simulink model "simulator_real"  (R2025b)
settings: Solver=ode15s  StartTime=0.0  StopTime=50  FixedStep=0.001  RelTol=1e-3
InitFcn:
  | run('rocket3d_params.m')
values from neighbouring files (symbols this model uses):
  A_e = pi*(d_e/2)^2    (= 0.000346360590058)    [rocket3d_params.m]
  A_rocket = pi*(d_rocket/2)^2    (= 0.006647610055)    [rocket3d_params.m]
  beta_poly = 1.31    [rocket3d_params.m]
  C_d_air = 0.90    (= 0.9)    [rocket3d_params.m]
  C_D_drag = 0.25    [rocket3d_params.m]
  C_d_water = 0.85    [rocket3d_params.m]
  CG_dry_body = [0.01289;  0.01855; -0.00576]    [rocket3d_params.m]
  CG_dry_Y = 0.01855    [rocket3d_params.m]
  CG_full_body = [0.01345; -0.10517; -0.00608]    [rocket3d_params.m]
  CG_full_Y = -0.10517    [rocket3d_params.m]
  D = q * A_rocket * Cd0    [aero_func.m]
  gamma_gas = 1.4    [rocket3d_params.m]
  I_dry_vec = [3.0e-3;  5.071e-4; 3.0e-3;  6.928e-7;  2.156e-6; -2.712e-6]    [rocket3d_params.m]
  I_full_vec = [1.1e-2;  1.0e-3;   1.1e-2;  3.14e-5;   2.234e-6; -1.994e-5]    [rocket3d_params.m]
  m_dry_i = 0.269    [rocket3d_params.m]
  m_empty = m_dry_i    (= 0.269)    [rocket3d_params.m]
  m_full = m_dry_i + m_water_0    (= 0.849)    [rocket3d_params.m]
  m_water_0 = 0.580    (= 0.58)    [rocket3d_params.m]
  N = round(t_sim/Ts)    [stability_margin_timehistory.m]
  P_atm = 101325    [rocket3d_params.m]
  P_i = 50*6894.75 + P_atm    (= 446062.5)    [rocket3d_params.m]
  R_gas = 287.05    [rocket3d_params.m]
  rho_air_ext = 1.225    [rocket3d_params.m]
  rho_water = 1000    [rocket3d_params.m]
  T_i = T_celsius + 273.15    (= 298.15)    [rocket3d_params.m]
  Ts = 0.001    [rocket3d_params.m]    (also in stability_margin_timehistory.m)
  V_bottle = 1.5e-3    (= 0.0015)    [rocket3d_params.m]
  V_gas_i = V_bottle - V_water_i    (= 0.00092)    [rocket3d_params.m]
  Y_CP_body = 0.160119 - 0.255    (= -0.094881)    [rocket3d_params.m]
undefined symbols (not defined in the file or in its folder): X, Y, Z
libraries: nesl_utility x14, sm_lib x10
settings Model: Creator=user  LastModifiedBy=user

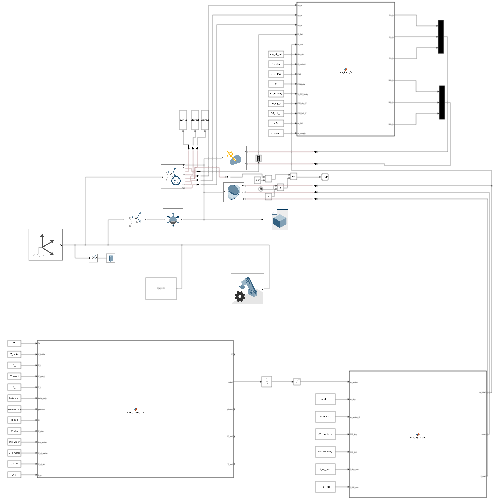
[thumbnail: Simulink's stored preview of the top-level diagram]
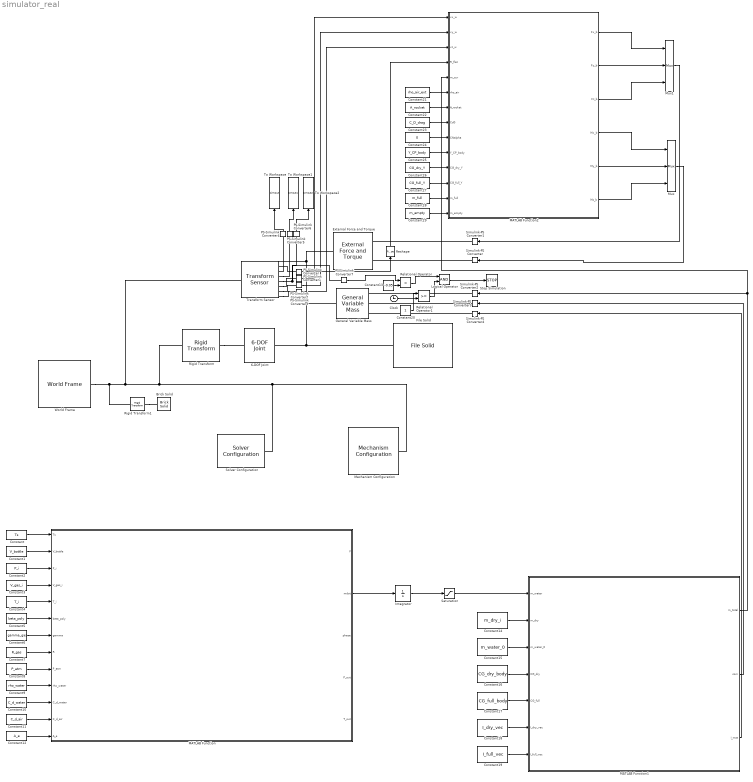
== system simulator_real ==
  6-DOF Joint : sm_lib/Joints/6-DOF Joint  JointMode=Normal  CompositeWrenchDir=FollowerOnBase  CompositeWrenchFrame=BaseFrame  SenseConstraintForce=off  SenseConstraintTorque=off  SenseTotalForce=off  SenseTotalTorque=off  PxPositionTargetSpecify=off  PxPositionTargetPriority=High  PxPositionTargetValue=0  PxPositionTargetValueUnits=m  PxVelocityTargetSpecify=off  PxVelocityTargetPriority=High  PxVelocityTargetValue=0  PxVelocityTargetValueUnits=m/s  PxEquilibriumPosition=0  PxEquilibriumPositionUnits=m  PxSpringStiffness=0  PxSpringStiffnessUnits=N/m  PxDampingCoefficient=0  PxDampingCoefficientUnits=N/(m/s)  PxLowerLimitSpecify=off  PxLowerLimitBound=-1  PxLowerLimitBoundUnits=m  PxLowerLimitStiffness=1e6  PxLowerLimitStiffnessUnits=N/m  PxLowerLimitDamping=1e3  PxLowerLimitDampingUnits=N/(m/s)  PxLowerLimitTransitionRegionWidth=1e-4  PxLowerLimitTransitionRegionWidthUnits=m  PxUpperLimitSpecify=off  PxUpperLimitBound=1  PxUpperLimitBoundUnits=m  PxUpperLimitStiffness=1e6  PxUpperLimitStiffnessUnits=N/m  PxUpperLimitDamping=1e3  PxUpperLimitDampingUnits=N/(m/s)  PxUpperLimitTransitionRegionWidth=1e-4  PxUpperLimitTransitionRegionWidthUnits=m  PxTorqueActuationMode=NoTorque  PxMotionActuationMode=ComputedMotion  PxSensePosition=off  PxSenseVelocity=off  PxSenseAcceleration=off  PxSenseTorqueForce=off  PxSenseLowerLimitTorqueForce=off  PxSenseUpperLimitTorqueForce=off  PyPositionTargetSpecify=off  PyPositionTargetPriority=High  PyPositionTargetValue=0  PyPositionTargetValueUnits=m  PyVelocityTargetSpecify=off  PyVelocityTargetPriority=High  PyVelocityTargetValue=0  PyVelocityTargetValueUnits=m/s  PyEquilibriumPosition=0  PyEquilibriumPositionUnits=m  PySpringStiffness=0  PySpringStiffnessUnits=N/m  PyDampingCoefficient=0  PyDampingCoefficientUnits=N/(m/s)  PyLowerLimitSpecify=off  PyLowerLimitBound=-1  PyLowerLimitBoundUnits=m  PyLowerLimitStiffness=1e6  PyLowerLimitStiffnessUnits=N/m  PyLowerLimitDamping=1e3  PyLowerLimitDampingUnits=N/(m/s)  PyLowerLimitTransitionRegionWidth=1e-4  PyLowerLimitTransitionRegionWidthUnits=m  PyUpperLimitSpecify=off  PyUpperLimitBound=1  PyUpperLimitBoundUnits=m  PyUpperLimitStiffness=1e6  PyUpperLimitStiffnessUnits=N/m  PyUpperLimitDamping=1e3  PyUpperLimitDampingUnits=N/(m/s)  PyUpperLimitTransitionRegionWidth=1e-4  PyUpperLimitTransitionRegionWidthUnits=m  PyTorqueActuationMode=NoTorque  PyMotionActuationMode=ComputedMotion  PySensePosition=off  PySenseVelocity=off  PySenseAcceleration=off  PySenseTorqueForce=off  PySenseLowerLimitTorqueForce=off  PySenseUpperLimitTorqueForce=off  PzPositionTargetSpecify=on  PzPositionTargetPriority=High  PzPositionTargetValue=0.3  PzPositionTargetValueUnits=m  PzVelocityTargetSpecify=off  PzVelocityTargetPriority=High  PzVelocityTargetValue=0  PzVelocityTargetValueUnits=m/s  PzEquilibriumPosition=0  PzEquilibriumPositionUnits=m  PzSpringStiffness=0  PzSpringStiffnessUnits=N/m  PzDampingCoefficient=0  PzDampingCoefficientUnits=N/(m/s)  PzLowerLimitSpecify=off  PzLowerLimitBound=-1  PzLowerLimitBoundUnits=m  PzLowerLimitStiffness=1e6  PzLowerLimitStiffnessUnits=N/m  PzLowerLimitDamping=1e3  PzLowerLimitDampingUnits=N/(m/s)  PzLowerLimitTransitionRegionWidth=1e-4  PzLowerLimitTransitionRegionWidthUnits=m  PzUpperLimitSpecify=off  PzUpperLimitBound=1  PzUpperLimitBoundUnits=m  PzUpperLimitStiffness=1e6  PzUpperLimitStiffnessUnits=N/m  PzUpperLimitDamping=1e3  PzUpperLimitDampingUnits=N/(m/s)  PzUpperLimitTransitionRegionWidth=1e-4  PzUpperLimitTransitionRegionWidthUnits=m  PzTorqueActuationMode=NoTorque  PzMotionActuationMode=ComputedMotion  PzSensePosition=off  PzSenseVelocity=off  PzSenseAcceleration=off  PzSenseTorqueForce=off  PzSenseLowerLimitTorqueForce=off  PzSenseUpperLimitTorqueForce=off  SphPositionTargetSpecify=off  SphPositionTargetPriority=High  SphPositionTargetRotationMethod=None  SphPositionTargetFollAlignAxisA=+X  SphPositionTargetBaseAlignAxisA=+Y  SphPositionTargetFollAlignAxisB=+Y  SphPositionTargetBaseAlignAxisB=+Z  SphPositionTargetRotationStandardAxis=+Z  SphPositionTargetRotationAngle=0  SphPositionTargetRotationAngleUnits=deg  SphPositionTargetRotationArbitraryAxis=[0 0 1]  SphPositionTargetRotationSequenceAxes=FollowerAxes  SphPositionTargetRotationSequence=XYX  SphPositionTargetRotationSequenceAngles=[0 0 0]  SphPositionTargetRotationSequenceAnglesUnits=deg  SphPositionTargetRotationMatrix=[1 0 0;0 1 0;0 0 1]  SphPositionTargetQuaternion=[1 0 0 0]  SphVelocityTargetSpecify=off  SphVelocityTargetPriority=High  SphVelocityTargetValue=[0 0 0]  SphVelocityTargetValueUnits=deg/s  SphVelocityTargetInFollowerFrame=on  SphEqPosRotationMethod=None  SphEqPosFollAlignAxisA=+X  SphEqPosBaseAlignAxisA=+Y  SphEqPosFollAlignAxisB=+Y  SphEqPosBaseAlignAxisB=+Z  SphEqPosRotationStandardAxis=+Z  SphEqPosRotationAngle=0  SphEqPosRotationAngleUnits=deg  SphEqPosRotationArbitraryAxis=[0 0 1]  SphEqPosRotationSequenceAxes=FollowerAxes  SphEqPosRotationSequence=XYX  SphEqPosRotationSequenceAngles=[0 0 0]  SphEqPosRotationSequenceAnglesUnits=deg  SphEqPosRotationMatrix=[1 0 0;0 1 0;0 0 1]  SphEqPosQuaternion=[1 0 0 0]  SphSpringStiffness=0  SphSpringStiffnessUnits=N*m/deg  SphDampingCoefficient=0  SphDampingCoefficientUnits=N*m/(deg/s)  SphLowerLimitSpecify=off  SphLowerLimitBound=15  SphLowerLimitBoundUnits=deg  SphLowerLimitStiffness=1e4  SphLowerLimitStiffnessUnits=N*m/deg  SphLowerLimitDamping=10  SphLowerLimitDampingUnits=N*m/(deg/s)  SphLowerLimitTransitionRegionWidth=0.1  SphLowerLimitTransitionRegionWidthUnits=deg  SphUpperLimitSpecify=off  SphUpperLimitBound=45  SphUpperLimitBoundUnits=deg  SphUpperLimitStiffness=1e4  SphUpperLimitStiffnessUnits=N*m/deg  SphUpperLimitDamping=10  SphUpperLimitDampingUnits=N*m/(deg/s)  SphUpperLimitTransitionRegionWidth=0.1  SphUpperLimitTransitionRegionWidthUnits=deg  SphTorqueActuationMode=NoTorque  SphActuateTorqueX=off  SphActuateTorqueY=off  SphActuateTorqueZ=off  SphActuateTorque=off  SphActuationFrame=BaseFrame  SphSensePosition=off  SphSenseVelocityX=off  SphSenseVelocityY=off  SphSenseVelocityZ=off  SphSenseVelocity=off  SphSenseAccelerationX=off  SphSenseAccelerationY=off  SphSenseAccelerationZ=off  SphSenseAcceleration=off  SphSenseLowerLimitTorqueMag=off  SphSenseUpperLimitTorqueMag=off  SphSensingFrame=BaseFrame
  Brick Solid : sm_lib/Body Elements/Brick Solid  BrickDimensions=[100, 0.0001, 100]  BrickDimensionsUnits=m  ExportEntireGeometry=off  InertiaType=Custom  BasedOnType=Density  Density=1000  DensityUnits=kg/m^3  Mass=1e6  MassUnits=kg  CenterOfMass=[0 0 0]  CenterOfMassUnits=m  MomentsOfInertia=[1e10 1e10 1e10]  MomentsOfInertiaUnits=kg*m^2  ProductsOfInertia=[0 0 0]  ProductsOfInertiaUnits=kg*m^2  GraphicType=FromGeometry  MarkerShape=Sphere  MarkerSize=10  GraphicVisPropType=SimpleVisualProperties  GraphicDiffuseColor=[0.5 0.5 0.5]  GraphicOpacity=1  GraphicSpecularColor=[0.5 0.5 0.5 1.0]  GraphicAmbientColor=[0.15 0.15 0.15 1.0]  GraphicEmissiveColor=[0.0 0.0 0.0 1.0]  GraphicShininess=75  DoExposeReferenceFrame=on  SerializedFrames=<Frames/>
  Clock : Clock
  Constant : Constant  Value=Ts
  Constant1 : Constant  Value=V_bottle
  Constant10 : Constant  Value=C_d_water
  Constant11 : Constant  Value=C_d_air
  Constant12 : Constant  Value=A_e
  Constant13 : Constant  Value=-0.05
  Constant14 : Constant  Value=m_dry_i
  Constant15 : Constant  Value=m_water_0
  Constant16 : Constant  Value=CG_dry_body
  Constant17 : Constant  Value=CG_full_body
  Constant18 : Constant  Value=I_dry_vec
  Constant19 : Constant  Value=I_full_vec
  Constant2 : Constant  Value=P_i
  Constant20 : Constant
  Constant21 : Constant  Value=rho_air_ext
  Constant22 : Constant  Value=A_rocket
  Constant23 : Constant  Value=C_D_drag
  Constant24 : Constant  Value=0
  Constant25 : Constant  Value=Y_CP_body
  Constant26 : Constant  Value=CG_dry_Y
  Constant27 : Constant  Value=CG_full_Y
  Constant28 : Constant  Value=m_full
  Constant29 : Constant  Value=m_empty
  Constant3 : Constant  Value=V_gas_i
  Constant4 : Constant  Value=T_i
  Constant5 : Constant  Value=beta_poly
  Constant6 : Constant  Value=gamma_gas
  Constant7 : Constant  Value=R_gas
  Constant8 : Constant  Value=P_atm
  Constant9 : Constant  Value=rho_water
  External Force and Torque : sm_lib/Forces and Torques/External Force and Torque  EnableForceX=off  EnableForceY=off  EnableForceZ=off  EnableForce=on  ForceResolutionFrame=AttachedFrame  EnableTorqueX=off  EnableTorqueY=off  EnableTorqueZ=off  EnableTorque=on  TorqueResolutionFrame=AttachedFrame
  File Solid : sm_lib/Body Elements/File Solid  ExtGeomFileName=C:\Users\user\Desktop\water_rocket_simulator\water_rocket_stp.stp  UnitType=Custom  ExtGeomFileUnits=mm  StepReaderType=HEX  ExportConvexHullGeometry=off  InertiaType=Custom  BasedOnType=DensityFromFile  Density=1000  DensityUnits=kg/m^3  Mass=0  MassUnits=kg  CenterOfMass=[0 0 0]  CenterOfMassUnits=m  MomentsOfInertia=[1e-12 1e-12 1e-12]  MomentsOfInertiaUnits=kg*m^2  ProductsOfInertia=[0 0 0]  ProductsOfInertiaUnits=kg*m^2  GraphicType=FromGeometry  MarkerShape=Sphere  MarkerSize=10  GraphicVisPropType=SimpleVisualProperties  GraphicDiffuseColor=[0.5 0.5 0.5]  GraphicOpacity=1  GraphicSpecularColor=[0.5 0.5 0.5 1.0]  GraphicAmbientColor=[0.15 0.15 0.15 1.0]  GraphicEmissiveColor=[0.0 0.0 0.0 1.0]  GraphicShininess=75  DoExposeReferenceFrame=on  SerializedFrames=<Frames/>
  General Variable Mass : sm_lib/Body Elements/Variable Mass/General Variable Mass  VariableInertiaType=Custom  MassType=TimeVarying  Mass=1  MassUnits=kg  CenterOfMassType=TimeVarying  CenterOfMass=[0 0 0]  CenterOfMassUnits=m  InertiaMatrixType=TimeVarying  MomentsOfInertia=[1 1 1]  MomentsOfInertiaUnits=kg*m^2  ProductsOfInertia=[0 0 0]  ProductsOfInertiaUnits=kg*m^2  GraphicType=InertiaEllipsoid  MarkerShape=Sphere  MarkerSize=10  GraphicVisPropType=SimpleVisualProperties  GraphicDiffuseColor=[0.5 0.5 0.5]  GraphicOpacity=1  GraphicSpecularColor=[0.5 0.5 0.5 1.0]  GraphicAmbientColor=[0.15 0.15 0.15 1.0]  GraphicEmissiveColor=[0.0 0.0 0.0 1.0]  GraphicShininess=75
  Integrator : Integrator  InitialCondition=m_water_0
  Logical Operator : Logic  AllPortsSameDT=off  OutDataTypeStr=boolean
  MATLAB Function : MATLAB Function  TreatAsAtomicUnit=on
  MATLAB Function1 : MATLAB Function  TreatAsAtomicUnit=on
  MATLAB Function2 : MATLAB Function  TreatAsAtomicUnit=on
  Mechanism Configuration : sm_lib/Utilities/Mechanism Configuration  UniformGravity=Constant  GravityVector=[0 0 -9.81]  GravityVectorUnits=m/s^2  LinearizationDelta=0.001  JointModeTransitionNonlinearIterations=2
  Mux : Mux  Inputs=3
  Mux1 : Mux  Inputs=3
  PS-Simulink Converter{,1..7} (8 alike) : nesl_utility/PS-Simulink Converter  PhysicalDomain=network_engine_domain  SubClassName=ps_output  LeftPortType=input  RightPortType=output  PseudoPeriodic=off  Frequencies=[]  VectorFormat=inherit  Unit=inherit  AffineConversion=off
  Relational Operator : RelationalOperator  Operator=<  OutDataTypeStr=boolean  RndMeth=Simplest  InputSameDT=off
  Relational Operator1 : RelationalOperator  OutDataTypeStr=boolean  RndMeth=Simplest  InputSameDT=off
  Reshape : Reshape  OutputDimensionality=Column vector (2-D)
  Rigid Transform : sm_lib/Frames and Transforms/Rigid Transform  RotationMethod=RotationMatrix  FollAlignAxisA=+X  BaseAlignAxisA=+Y  FollAlignAxisB=+Y  BaseAlignAxisB=+Z  RotationStandardAxis=+Z  RotationAngle=0  RotationAngleUnits=deg  RotationArbitraryAxis=[0 0 1]  RotationSequenceAxes=FollowerAxes  RotationSequence=XYX  RotationSequenceAngles=[0 0 0]  RotationSequenceAnglesUnits=deg  RotationMatrix=R_init  Quaternion=[1 0 0 0]  TranslationMethod=Cartesian  TranslationCartesianOffset=[0 0 0]  TranslationCartesianOffsetUnits=m  TranslationStandardAxis=+Z  TranslationStandardOffset=0  TranslationStandardOffsetUnits=m  TranslationROffset=0  TranslationROffsetUnits=m  TranslationThetaOffset=0  TranslationThetaOffsetUnits=deg  TranslationZOffset=0  TranslationZOffsetUnits=m
  Rigid Transform1 : sm_lib/Frames and Transforms/Rigid Transform  RotationMethod=None  FollAlignAxisA=+X  BaseAlignAxisA=+Y  FollAlignAxisB=+Y  BaseAlignAxisB=+Z  RotationStandardAxis=+Z  RotationAngle=0  RotationAngleUnits=deg  RotationArbitraryAxis=[0 0 1]  RotationSequenceAxes=FollowerAxes  RotationSequence=XYX  RotationSequenceAngles=[0 0 0]  RotationSequenceAnglesUnits=deg  RotationMatrix=[1 0 0;0 1 0;0 0 1]  Quaternion=[1 0 0 0]  TranslationMethod=Cartesian  TranslationCartesianOffset=[0 0 0]  TranslationCartesianOffsetUnits=m  TranslationStandardAxis=+Z  TranslationStandardOffset=0  TranslationStandardOffsetUnits=m  TranslationROffset=0  TranslationROffsetUnits=m  TranslationThetaOffset=0  TranslationThetaOffsetUnits=deg  TranslationZOffset=0  TranslationZOffsetUnits=m
  Saturation : Saturate  UpperLimit=m_water_0  LowerLimit=0
  Simulink-PS Converter{,1..4} (5 alike) : nesl_utility/Simulink-PS Converter  PhysicalDomain=network_engine_domain  SubClassName=ps_input  LeftPortType=input  RightPortType=output  PseudoPeriodic=off  Frequencies=[]  NoiseDistribution=none  NoiseParameters=[]  Unit=1  AffineConversion=off  FilteringAndDerivatives=provide  SimscapeFilterOrder=1  InputFilterTimeConstant=0.001  UdotUserProvided=0
  Solver Configuration : nesl_utility/Solver Configuration  PhysicalDomain=network_engine_domain  SubClassName=solver  LeftPortType=input  RightPortType=generic  Tones=[]  Harmonics=[]  SimulateNoise=off  Profile=off  UseLocalSampling=off  EnableSwitchedLinearOptims=on  FrequencyDomain=off  UseCCode=off  RelTol=0.001  AbsTol=0.001  MinStep=1e-09  ToWorkspace=off  RevertToSquareIcSolve=off  NumHomotopyIterations=100  PhasorMode=off  PhasorModeNumHarmonics=1  ConsistencySolver=NEWTON_XTOL_AFTER_FTOL  IndexReductionMethod=DerivativeReplacement  DoDC=off  ResidualTolerance=1e-09  ConsistencyTolSource=GLOBAL  ConsistencyAbsTol=0.001  ConsistencyRelTol=0.001  ConsistencyTolFactor=0.001  UseLocalSolver=off  LocalSolverChoice=NE_BACKWARD_EULER_ADVANCER  ResolveIndetEquations=on  FunctionEvalNumThread=1  LocalSolverSampleTime=0.001  DoFixedCost=off  MaxNonlinIter=3  MaxModeIter=2  ComputeImpulses=off  ImpulseIterations=2  LinearAlgebra=auto  LinearAlgebraNumThread=0  EquationFormulation=NE_TIME_EF  DelaysMemoryBudget=1024  AutomaticFiltering=on  FilteringTimeConstant=0.001  PartitionStorageMethod=AS_NEEDED  PartitionMemoryBudget=1024  PartitionMethod=ROBUST  MultibodyUseLocalSolver=off  MultibodyLocalSolverChoice=ODE1  MultibodyLocalSolverSampleTime=0.001
  Stop Simulation : Stop
  To Workspace : ToWorkspace  VariableName=simout  SaveFormat=Timeseries  SampleTime=-1
  To Workspace1 : ToWorkspace  VariableName=simout1  SaveFormat=Timeseries  SampleTime=-1
  To Workspace2 : ToWorkspace  VariableName=simout2  SaveFormat=Timeseries  SampleTime=-1
  Transform Sensor : sm_lib/Frames and Transforms/Transform Sensor  MeasurementFrame=World  RotationSequence=XYX  SenseAngle=off  SenseAxis=off  SenseQ=off  SenseR=on  SenseRotationSequence=off  SenseOmegaX=off  SenseOmegaY=off  SenseOmegaZ=off  SenseOmega=off  SenseQDot=off  SenseRDot=off  SenseRotationSequenceDot=off  SenseAlphaX=off  SenseAlphaY=off  SenseAlphaZ=off  SenseAlpha=off  SenseQDDot=off  SenseRDDot=off  SenseX=on  SenseY=on  SenseZ=on  SenseXYZ=off  SenseRad=off  SenseAzim=off  SenseDist=off  SenseInc=off  SenseXDot=on  SenseYDot=on  SenseZDot=on  SenseXYZDot=off  SenseRadDot=off  SenseAzimDot=off  SenseDistDot=off  SenseIncDot=off  SenseXDDot=off  SenseYDDot=off  SenseZDDot=off  SenseXYZDDot=off  SenseRadDDot=off  SenseAzimDDot=off  SenseDistDDot=off  SenseIncDDot=off
  World Frame : sm_lib/Frames and Transforms/World Frame
  wires:
  Constant9/1 -> MATLAB Function/10(rho_water)
  Constant2/1 -> MATLAB Function/3(P_i)
  Constant1/1 -> MATLAB Function/2(V_bottle)
  Constant11/1 -> MATLAB Function/12(C_d_air)
  Constant4/1 -> MATLAB Function/5(T_i)
  Constant7/1 -> MATLAB Function/8(R)
  Constant5/1 -> MATLAB Function/6(beta_poly)
  Constant12/1 -> MATLAB Function/13(A_e)
  Constant10/1 -> MATLAB Function/11(C_d_water)
  Constant3/1 -> MATLAB Function/4(V_gas_i)
  Constant/1 -> MATLAB Function/1(Ts)
  Constant8/1 -> MATLAB Function/9(P_atm)
  Constant6/1 -> MATLAB Function/7(gamma)
  MATLAB Function/2(mdot) -> Integrator/1
  Integrator/1 -> Saturation/1
  Constant14/1 -> MATLAB Function1/2(m_dry)
  Constant15/1 -> MATLAB Function1/3(m_water_0)
  Constant16/1 -> MATLAB Function1/4(CG_dry)
  Constant17/1 -> MATLAB Function1/5(CG_full)
  Constant18/1 -> MATLAB Function1/6(I_dry_vec)
  Constant19/1 -> MATLAB Function1/7(I_full_vec)
  PS-Simulink Converter/1 -> Reshape/1
  Reshape/1 -> MATLAB Function2/4(R_flat)
  PS-Simulink Converter1/1 -> MATLAB Function2/1(vx_w)
  PS-Simulink Converter2/1 -> MATLAB Function2/2(vy_w)
  PS-Simulink Converter3/1 -> MATLAB Function2/3(vz_w)
  Constant21/1 -> MATLAB Function2/6(rho_air)
  Constant22/1 -> MATLAB Function2/7(A_rocket)
  Constant23/1 -> MATLAB Function2/8(Cd0)
  Constant24/1 -> MATLAB Function2/9(CNalpha)
  Constant25/1 -> MATLAB Function2/10(Y_CP_body)
  Constant26/1 -> MATLAB Function2/11(CG_dry_Y)
  Constant27/1 -> MATLAB Function2/12(CG_full_Y)
  Constant28/1 -> MATLAB Function2/13(m_full)
  Constant29/1 -> MATLAB Function2/14(m_empty)
  Saturation/1 -> MATLAB Function1/1(m_water)
  MATLAB Function1/1(m_total) -> MATLAB Function2/5(m_cur), Simulink-PS Converter2/1
  MATLAB Function2/4(Mx_b) -> Mux/1
  MATLAB Function2/5(My_b) -> Mux/2
  MATLAB Function2/6(Mz_b) -> Mux/3
  Mux/1 -> Simulink-PS Converter/1
  MATLAB Function2/1(Fx_b) -> Mux1/1
  MATLAB Function2/2(Fy_b) -> Mux1/2
  MATLAB Function2/3(Fz_b) -> Mux1/3
  Mux1/1 -> Simulink-PS Converter1/1
  MATLAB Function1/2(com) -> Simulink-PS Converter3/1
  MATLAB Function1/3(I_mat) -> Simulink-PS Converter4/1
  PS-Simulink Converter4/1 -> To Workspace/1
  PS-Simulink Converter5/1 -> To Workspace1/1
  PS-Simulink Converter6/1 -> To Workspace2/1
  Constant13/1 -> Relational Operator/2
  PS-Simulink Converter7/1 -> Relational Operator/1
  Relational Operator/1 -> Logical Operator/1
  Logical Operator/1 -> Stop Simulation/1
  Clock/1 -> Relational Operator1/1
  Relational Operator1/1 -> Logical Operator/2
  Constant20/1 -> Relational Operator1/2
  connections:
  World Frame/RConn1 -- Rigid Transform1/LConn1 -- Rigid Transform/LConn1 -- Solver Configuration/RConn1 -- Mechanism Configuration/RConn1 -- Transform Sensor/LConn1
  File Solid/RConn1 -- 6-DOF Joint/RConn1 -- General Variable Mass/RConn1 -- External Force and Torque/RConn1 -- Transform Sensor/RConn1
  Rigid Transform/RConn1 -- 6-DOF Joint/LConn1
  PS-Simulink Converter/LConn1 -- Transform Sensor/RConn2
  Transform Sensor/RConn6 -- PS-Simulink Converter1/LConn1
  Transform Sensor/RConn7 -- PS-Simulink Converter2/LConn1
  Transform Sensor/RConn8 -- PS-Simulink Converter3/LConn1
  Simulink-PS Converter/RConn1 -- External Force and Torque/LConn2
  Simulink-PS Converter1/RConn1 -- External Force and Torque/LConn1
  Simulink-PS Converter2/RConn1 -- General Variable Mass/LConn1
  Simulink-PS Converter3/RConn1 -- General Variable Mass/LConn2
  Simulink-PS Converter4/RConn1 -- General Variable Mass/LConn3
  Transform Sensor/RConn3 -- PS-Simulink Converter4/LConn1
  Transform Sensor/RConn4 -- PS-Simulink Converter5/LConn1
  Transform Sensor/RConn5 -- PS-Simulink Converter7/LConn1 -- PS-Simulink Converter6/LConn1
  Rigid Transform1/RConn1 -- Brick Solid/RConn1

== matlab function simulator_real/MATLAB Function1 ==
  data: m_water input; m_total output; m_dry input; m_water_0 input; CG_dry input; CG_full input; I_dry_vec input; I_full_vec input; com output; I_mat output
function [m_total, com, I_mat] = mass_cg_inertia(m_water, ...
        m_dry, m_water_0, CG_dry, CG_full, I_dry_vec, I_full_vec)
%#codegen
% 현재 물 질량에 따라 전체 질량·무게중심·관성 보간
% 입력
%   m_water   : 현재 물 질량 [kg] (Integrator 출력)
%   m_dry     : 건조 질량 [kg]
%   m_water_0 : 초기 물 질량 [kg]
%   CG_dry    : 건조 CG (CATIA 글로벌 좌표) [3×1, m]
%   CG_full   : 만수 CG (CATIA 글로벌 좌표) [3×1, m]
%   I_dry_vec : 건조 관성 [6×1, kg·m²] [Ixx;Iyy;Izz;Ixy;Ixz;Iyz]
%   I_full_vec: 만수 관성 [6×1, kg·m²]
% 출력
%   m_total   : 전체 질량 [kg]
%   com       : 현재 CG (body frame) [3×1, m]
%   I_vec     : 현재 관성텐서 [6×1, kg·m²]

frac = max(0.0, min(1.0, m_water / max(m_water_0, 1e-9)));

m_total = m_dry + m_water;
com     = CG_dry + frac * (CG_full - CG_dry);
Iv = I_dry_vec + frac * (I_full_vec - I_dry_vec);
I_mat = [Iv(1), Iv(4), Iv(5); ...
         Iv(4), Iv(2), Iv(6); ...
         Iv(5), Iv(6), Iv(3)];

== matlab function simulator_real/MATLAB Function ==
  data: Ts input; F output; V_bottle input; P_i input; V_gas_i input; T_i input; beta_poly input; gamma input; R input; P_atm input; rho_water input; C_d_water input; C_d_air input; A_e input; mdot output; phase output; P_out output; T_out output
function [F, mdot, phase, P_out, T_out] = thrust_phase_func(Ts, ...
        V_bottle, P_i, V_gas_i, T_i, beta_poly, gamma, R, P_atm, ...
        rho_water, C_d_water, C_d_air, A_e)
%#codegen
% 물로켓 추력 + 질량유량 계산
% (기존 2D 스크립트의 phase 1~3 while문 로직을 한 스텝짜리 함수로 이식)
%
% Simulink "MATLAB Function" 블록에 이 코드를 그대로 붙여넣고,
% 입력은 전부 rocket3d_params.m 의 값을 Constant 블록으로 연결하세요.
% (Ts만 샘플타임이고 나머지는 고정 파라미터입니다.)
%
% 출력
%   F     : 노즐 추력 [N]
%   mdot  : 추진제(물+공기) 질량유량 [kg/s] (분출이므로 음수)
%   phase : 현재 단계 (1=물 분출, 2=공기 분출, 3=탄도비행)
%   P_out, T_out : 내부 압력[Pa] / 온도[K] (로깅·디버깅용)

persistent V_gas P T phase_s P_phase2_i T_phase2_i

if isempty(V_gas)
    V_gas      = V_gas_i;
    P          = P_i;
    T          = T_i;
    phase_s    = uint8(1);
    P_phase2_i = P_i;
    T_phase2_i = T_i;
end

F = 0; mdot = 0;

switch phase_s
    case 1   % 물 분출 (폴리트로픽 압축공기 팽창)
        P = P_i * (V_gas_i / V_gas)^beta_poly;
        if P > P_atm
            v_e  = C_d_water * sqrt(2*(P - P_atm)/rho_water);
            F    = 2 * C_d_water^2 * A_e * (P - P_atm);
            mdot = -rho_water * A_e * v_e;
            V_gas = V_gas + A_e * v_e * Ts;
            if V_gas >= V_bottle
                V_gas      = V_bottle;
                phase_s    = uint8(2);
                P_phase2_i = P;
                T_phase2_i = T_i * (P / P_i)^((beta_poly - 1)/beta_poly);
                T = T_phase2_i;
            end
        else
            phase_s = uint8(2);
        end

    case 2   % 공기 분출 (단열 팽창, choked/subsonic 판정)
        if P > P_atm * 1.01
            T = T_phase2_i * (P / P_phase2_i)^((gamma - 1)/gamma);
            P_crit = 1.893 * P_atm;
            if P >= P_crit
                P_exit   = P * (2/(gamma+1))^(gamma/(gamma-1));
                T_exit   = T * (2/(gamma+1));
                v_exit   = sqrt(gamma * R * T_exit);
                rho_exit = P_exit / (R * T_exit);
                m_mag    = C_d_air * A_e * rho_exit * v_exit;
                F        = m_mag * v_exit + (P_exit - P_atm) * A_e;
                dP_dt    = -(C_d_air*A_e*gamma*P/V_bottle) * ...
                            sqrt(gamma*R*T*(2/(gamma+1))^((gamma+1)/(gamma-1)));
            else
                P_exit   = P_atm;
                v_exit   = sqrt((2*gamma*R*T/(gamma-1)) * (1 - (P_atm/P)^((gamma-1)/gamma)));
                T_exit   = T * (P_atm/P)^((gamma-1)/gamma);
                rho_exit = P_atm / (R * T_exit);
                m_mag    = C_d_air * A_e * rho_exit * v_exit;
                F        = m_mag * v_exit;
                term1 = (P_atm/P)^(2/gamma);
                term2 = (P_atm/P)^((gamma+1)/gamma);
                if term1 > term2
                    dP_dt = -(C_d_air*A_e*gamma*P/V_bottle) * ...
                             sqrt((2*gamma*R*T/(gamma-1)) * (term1 - term2));
                else
                    dP_dt = 0;
                end
            end
            mdot = -m_mag;
            P = P + dP_dt * Ts;
        else
            phase_s = uint8(3);
            P = P_atm;
        end

    case 3   % 탄도비행 (추력 없음)
    P = P_atm; F = 0; mdot = 0;
    k_heat = 5;                          % 대기와의 열교환 계수 (원본과 동일)
    T = T_i + (T - T_i) * exp(-k_heat*Ts);
end

phase = double(phase_s);
P_out = P;
T_out = T;
end

== matlab function simulator_real/MATLAB Function2 ==
  data: vx_w input; Fx_b output; vy_w input; vz_w input; R_flat input; m_cur input; rho_air input; A_rocket input; Cd0 input; CNalpha input; Y_CP_body input; CG_dry_Y input; CG_full_Y input; m_full input; m_empty input; Fy_b output; Fz_b output; Mx_b output; My_b output; Mz_b output
function [Fx_b, Fy_b, Fz_b, Mx_b, My_b, Mz_b] = aero_func_3d(...
        vx_w, vy_w, vz_w, R_flat, m_cur, ...
        rho_air, A_rocket, Cd0, CNalpha, ...
        Y_CP_body, CG_dry_Y, CG_full_Y, m_full, m_empty)
%#codegen
% 3D 공력 계산 (CATIA 기체축: Y = 동체 종축, 노즈콘 방향 = +Y)
%
% 입력
%   vx_w, vy_w, vz_w : Transform Sensor 출력 속도 [m/s] (World frame)
%   R_flat           : Transform Sensor 출력 회전행렬 [9×1, column-major]
%                      body→world 변환: v_world = R * v_body
%   m_cur            : 현재 전체 질량 [kg]
%   Y_CP_body        : CP의 CATIA Gy 좌표 [m] (= nosecone_tip_Y - x_CP)
%   CG_dry_Y / _full_Y : 건조/만수 CG의 CATIA Gy 좌표 [m]
% 출력
%   Fx_b~Fz_b : 기체축 힘 [N]  (External Force and Torque 입력)
%   Mx_b~Mz_b : 기체축 모멘트 [N·m]

R = reshape(R_flat, 3, 3);              % body→world 3×3
v_body = R' * [vx_w; vy_w; vz_w];     % world→body 속도 변환

u   = v_body(1);   % body X
v_Y = v_body(2);   % body Y (종축)
w   = v_body(3);   % body Z

V = sqrt(u^2 + v_Y^2 + w^2);

if V < 1e-3
    Fx_b=0; Fy_b=0; Fz_b=0; Mx_b=0; My_b=0; Mz_b=0;
    return
end

q = 0.5 * rho_air * V^2;

%% 축방향 항력 (속도 반대 방향)
D    = q * A_rocket * Cd0;
Fx_b = -D * (u  /V);
Fy_b = -D * (v_Y/V);
Fz_b = -D * (w  /V);

%% 받음각 / 옆미끄럼각 (기체 Y축 기준)
alpha_p = atan2(w,   v_Y);   % 피치 받음각
alpha_y = atan2(u,   v_Y);   % 요 옆미끄럼각

%% Barrowman 법선력
N_pitch = q * A_rocket * CNalpha * alpha_p;
N_yaw   = q * A_rocket * CNalpha * alpha_y;
Fz_b = Fz_b + N_pitch;
Fx_b = Fx_b + N_yaw;

%% 현재 CG의 Y 좌표 보간
frac   = (m_cur - m_empty) / max(m_full - m_empty, 1e-9);
frac   = max(0.0, min(1.0, frac));
CG_Y   = CG_dry_Y + frac * (CG_full_Y - CG_dry_Y);

%% CP-CG 모멘트 (r = CP - CG, 기체 Y축 방향)
r_Y = Y_CP_body - CG_Y;   % 음수 = CP가 CG보다 -Y(뒤쪽) = 안정

%  r × F:  r=[0;r_Y;0], F_pitch=[0;0;N_pitch] → Mx = r_Y*N_pitch
%           r=[0;r_Y;0], F_yaw =[N_yaw;0;0]   → Mz = -r_Y*N_yaw
Mx_b = r_Y * N_pitch;
My_b = 0;
Mz_b = -r_Y * N_yaw;
